simulink model "Lab_6_Task_3"  (R2022b)
settings: Solver=VariableStepAuto  StartTime=0.0  StopTime=10.0  MaxStep=0.01  RelTol=1e-3
settings Model: Creator=Azlaan  LastModifiedBy=Azlaan

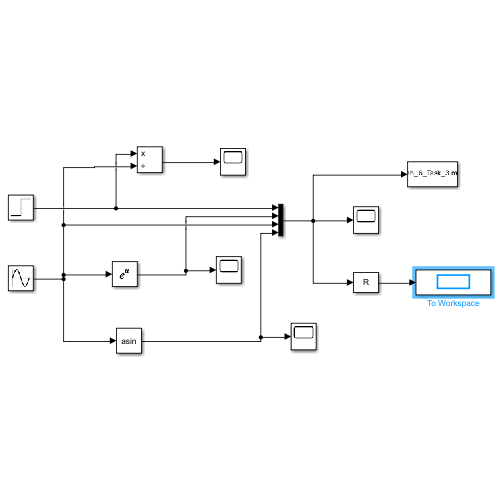
[thumbnail: Simulink's stored preview of the top-level diagram]
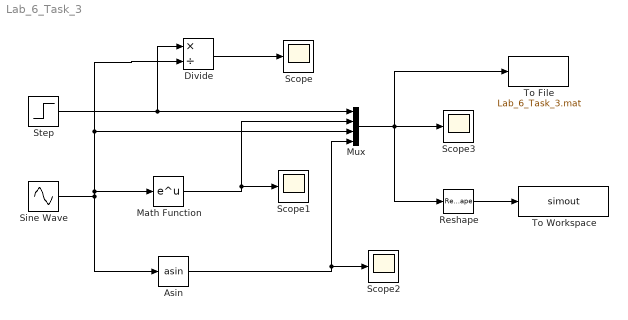
== system Lab_6_Task_3 ==
  Asin : Trigonometry  Operator=asin
  Divide : Product  Inputs=*/
  Math Function : Math
  Mux : Mux
  Reshape : Reshape  OutputDimensionality=Customize  OutputDimensions=[2,2]
  Scope{,1..3} (4 alike) : Scope
  Sine Wave : Sin  SampleTime=0
  Step : Step  SampleTime=0
  To File : ToFile  Filename=Lab_6_Task_3.mat  SaveFormat=Timeseries
  To Workspace : ToWorkspace  VariableName=simout  SampleTime=-1
  wires:
  Divide/1 -> Scope/1
  Sine Wave/1 -> Math Function/1, Mux/3, Divide/2, Asin/1
  Step/1 -> Mux/1, Divide/1
  Math Function/1 -> Scope1/1, Mux/2
  Asin/1 -> Scope2/1, Mux/4
  Mux/1 -> To File/1, Scope3/1, Reshape/1
  Reshape/1 -> To Workspace/1
